simulink model "MdSWReqChk"  (R2024b)
settings: Solver=FixedStepDiscrete  StartTime=0.0  StopTime=10.0  FixedStep=0.01  RelTol=1e-3
undefined symbols (not defined in the file or in its folder): ChkBsyBitArray4s, ChkBsyBitArray6s7s, KeSMSAutoEZEFwdBkwdPosEna_Val, KeSMSuButtonLongPressedThrshldTm_Val, KeSMSuMdNum4s_Val, KeSMSuMdNum6s7s_Val, SetBsyBitArray4s, SetEnBitArray4s
libraries: simulink x16, RspLib x14
(part 1 of 3)
settings Model: Creator=sn2xws  LastModifiedBy=sn55gm
settings Model: ModifiedHistory=|
  | 2023.8.1 CR401790  增加模式21-26的请求
  | V2.1.0
  | 2023.9.18 bug 542961符号方向反了，<= 改为>=
  | V2.3.0
  | 2023.12.28  迎宾向后，条件改为或
  | 2024.7.11 V3.0.0 557模式流程V1.9
  | 2024.8.15 V3.0.1 打断逻辑更新
  | 2024.8.19 V3.0.2 Md30 Md31临时关闭
  | 2024.9.2 V3.0.3 v3.0.1需求共存逻辑更新
  | 2024.9.26 V3.0.4 bsybitall 不使用的模式去除Md8
  | 2024.10.15 V3.0.5 增加Md57 Md58
  | 2024.11.5 V3.0.6 对req做跳变1判断
  | 2024.12.5 V3.0.7 Md8与Md30，md31应可以共存
  | 2024.12.19 V3.0.8 BUG 963441 Md9 与Md11不共存问题
  | 2024.12.19 V3.0.9 BUG 963459 Md53 与Md31不共存问题（NotUsedMode值错误，bsyall不看notusedmode）
  | 2024.12.24 V3.1.0 BUG 964134 VIPALL LUGALL VIPEXITALL模式可以单侧打断，只看剩余运行模式与其他模式共存的逻辑
  | 2024.12.25 V3.1.1 VIPRbsy应增加7sLUGR
  | 25.6.28 V3.13.0 新增大记忆模式MD61 MD62
  | 25.7.11 V3.13.1 md61 md62请求连反
settings SolverCC: AlgebraicLoopSolver=TrustRegion
settings DataIOCC: SaveFormat=StructureWithTime  ReturnWorkspaceOutputs=off
settings OptimizationCC: DefaultParameterBehavior=Inlined  EnhancedBackFolding=on  PassReuseOutputArgsAs=Individual arguments  ZeroExternalMemoryAtStartup=off  ZeroInternalMemoryAtStartup=off  OptimizeBlockOrder=speed  DifferentSizesBufferReuse=on  OptimizationCustomize=off  EfficientTunableParamExpr=on
settings DebuggingCC: ParameterTunabilityLossMsg=error  UnconnectedInputMsg=warning  UnconnectedOutputMsg=warning  UnconnectedLineMsg=warning  ArithmeticOperatorsInVariantConditions=warning
settings ModelReferenceCC: EnableRefExpFcnMdlSchedulingChecks=on  ModelReferenceNumInstancesAllowed=Single
settings SFSimCC: MATLABDynamicMemAlloc=off  CustomCodeUndefinedFunction=UseInterfaceOnly
settings RTWCC: Description=AUTOSAR  SystemTargetFile=autosar.tlc  GenCodeOnly=on  TemplateMakefile=ert_default_tmf  GenerateReport=on  IncludeHyperlinkInReport=on  LaunchReport=on  DataTypeReplacement=CDataTypesFixedWidth  GenerateTraceInfo=on  GenerateTraceReport=on  GenerateTraceReportSl=on  GenerateTraceReportSf=on  GenerateTraceReportEml=on  GenerateCodeMetricsReport=on  GPUComputeCapability=3.5
settings CodeAppCC: ForceParamTrailComments=on  IgnoreCustomStorageClasses=off  OperatorAnnotations=on  SimulinkDataObjDesc=on  SFDataObjDesc=on  InsertBlockDesc=on
settings STFCustomTargetCC: TargetLangStandard=C99 (ISO)  MultiwordLength=256  ParMdlRefBuildCompliant=on  CompOptLevelCompliant=on  IncludeMdlTerminateFcn=off  CombineOutputUpdateFcns=on  SuppressErrorStatus=on  ERTCustomFileBanners=on  SupportNonFinite=off  SupportComplex=off  SupportContinuousTime=off  SupportNonInlinedSFcns=off  RemoveResetFunc=on  MATLABClassNameForMDSCustomization=Simulink.SoftwareTarget.ERTCustomization  AutosarCompliant=on  UseToolchainInfoCompliant=on  LookupTableObjectStructAxisOrder=2,1,3,4,...  LUTObjectStructOrderEvenSpacing=Size,Table,Breakpoints  SystemTargetFile=autosar.tlc
settings ERTTargetCC: TargetLangStandard=C99 (ISO)  ConcurrentExecutionCompliant=off  IncludeMdlTerminateFcn=off  SuppressErrorStatus=on  SupportNonFinite=off  SupportComplex=off  ModelStepFunctionPrototypeControlCompliant=off  CPPClassGenCompliant=off  AutosarCompliant=on  LookupTableObjectStructAxisOrder=2,1,3,4,...  LUTObjectStructOrderEvenSpacing=Size,Table,Breakpoints  ERTCustomFileTemplate=example_file_process.tlc  ERTFilePackagingFormat=Compact  BooleanTrueId=TRUE  BooleanFalseId=FALSE  DynamicArrayContainerType=coder::array

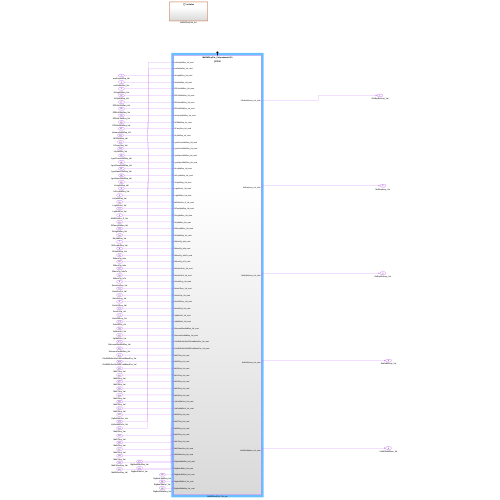
[thumbnail: Simulink's stored preview of the top-level diagram]
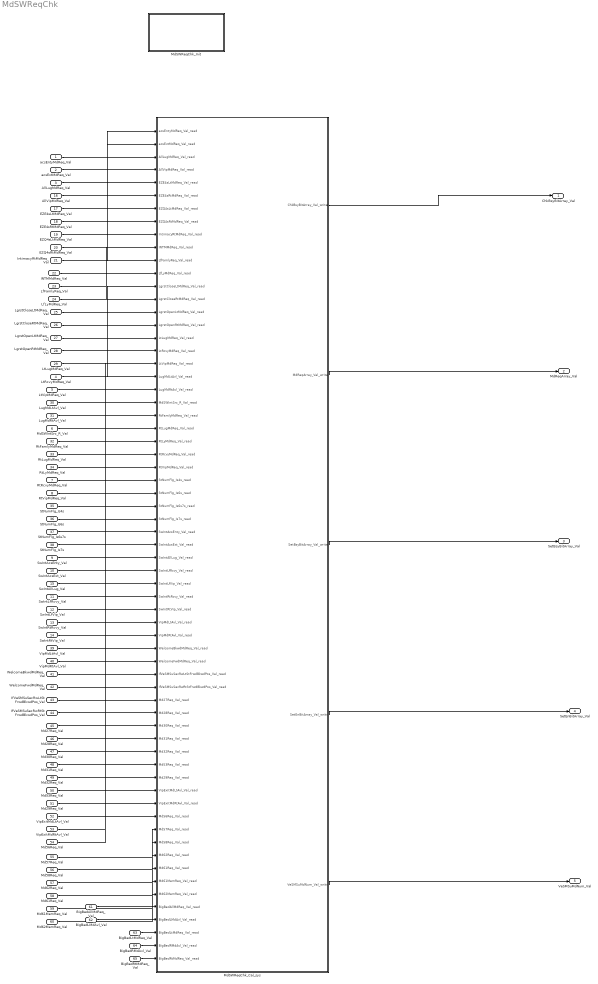
== system MdSWReqChk ==
  acsEntyMdReq_Val : Inport  OutDataTypeStr=boolean  PortDimensions=1
  acsExtMdReq_Val : Inport  Port=2  OutDataTypeStr=boolean  PortDimensions=1
  AllLugMdReq_Val : Inport  Port=3  OutDataTypeStr=boolean  PortDimensions=1
  LtRcvyMdReq_Val : Inport  Port=4  OutDataTypeStr=boolean  PortDimensions=1
  LtVipMdReq_Val : Inport  Port=5  OutDataTypeStr=boolean  PortDimensions=1
  MdSWIntSrc_R_Val : Inport  Port=6  OutDataTypeStr=uint16  PortDimensions=1
  RtRcvyMdReq_Val : Inport  Port=7  OutDataTypeStr=boolean  PortDimensions=1
  RtVipMdReq_Val : Inport  Port=8  OutDataTypeStr=boolean  PortDimensions=1
  SwIntAcsEnty_Val : Inport  Port=9  OutDataTypeStr=IntEnable  PortDimensions=1
  SwIntAcsExt_Val : Inport  Port=10  OutDataTypeStr=IntEnable  PortDimensions=1
  SwIntLfRcvy_Val : Inport  Port=11  OutDataTypeStr=IntEnable  PortDimensions=1
  SwIntLfVip_Val : Inport  Port=12  OutDataTypeStr=IntEnable  PortDimensions=1
  SwIntRtRcvy_Val : Inport  Port=13  OutDataTypeStr=IntEnable  PortDimensions=1
  SwIntRtVip_Val : Inport  Port=14  OutDataTypeStr=IntEnable  PortDimensions=1
  SwIntAllLug_Val : Inport  Port=15  OutDataTypeStr=IntEnable  PortDimensions=1
  AllVipMdReq_Val : Inport  Port=16  OutDataTypeStr=boolean  PortDimensions=1
  EZE4sLtMdReq_Val : Inport  Port=17  OutDataTypeStr=boolean  PortDimensions=1
  EZE4sRtMdReq_Val : Inport  Port=18  OutDataTypeStr=boolean  PortDimensions=1
  EZQ4sLtMdReq_Val : Inport  Port=19  OutDataTypeStr=boolean  PortDimensions=1
  EZQ4sRtMdReq_Val : Inport  Port=20  OutDataTypeStr=boolean  PortDimensions=1
  IntimacyRtMdReq_Val : Inport  Port=21  OutDataTypeStr=boolean  PortDimensions=1
  INTMMdReq_Val : Inport  Port=22  OutDataTypeStr=boolean  PortDimensions=1
  LfFamlyReq_Val : Inport  Port=23  OutDataTypeStr=boolean  PortDimensions=1
  LfLyMdReq_Val : Inport  Port=24  OutDataTypeStr=boolean  PortDimensions=1
  LgrstCloseLtMdReq_Val : Inport  Port=25  OutDataTypeStr=boolean  PortDimensions=1
  LgrstCloseRtMdReq_Val : Inport  Port=26  OutDataTypeStr=boolean  PortDimensions=1
  LgrstOpenLtMdReq_Val : Inport  Port=27  OutDataTypeStr=boolean  PortDimensions=1
  LgrstOpenRtMdReq_Val : Inport  Port=28  OutDataTypeStr=boolean  PortDimensions=1
  LtLugMdReq_Val : Inport  Port=29  OutDataTypeStr=boolean  PortDimensions=1
  LugMdLtAvl_Val : Inport  Port=30  OutDataTypeStr=boolean  PortDimensions=1
  LugMdRtAvl_Val : Inport  Port=31  OutDataTypeStr=boolean  PortDimensions=1
  RtFamlyMdReq_Val : Inport  Port=32  OutDataTypeStr=boolean  PortDimensions=1
  RtLugMdReq_Val : Inport  Port=33  OutDataTypeStr=boolean  PortDimensions=1
  RtLyMdReq_Val : Inport  Port=34  OutDataTypeStr=boolean  PortDimensions=1
  StNumFlg_Is4s : Inport  Port=35  OutDataTypeStr=boolean  PortDimensions=1
  StNumFlg_Is6s : Inport  Port=36  OutDataTypeStr=boolean  PortDimensions=1
  StNumFlg_Is6s7s : Inport  Port=37  OutDataTypeStr=boolean  PortDimensions=1
  StNumFlg_Is7s : Inport  Port=38  OutDataTypeStr=boolean  PortDimensions=1
  VipMdLtAvl_Val : Inport  Port=39  OutDataTypeStr=boolean  PortDimensions=1
  VipMdRtAvl_Val : Inport  Port=40  OutDataTypeStr=boolean  PortDimensions=1
  WelcomeBkwdMdReq_Val : Inport  Port=41  OutDataTypeStr=boolean  PortDimensions=1
  WelcomeFwdMdReq_Val : Inport  Port=42  OutDataTypeStr=boolean  PortDimensions=1
  IfVeSMSuSecRwLtStFrwdBkwdPos_Val : Inport  Port=43  OutDataTypeStr=uint16  PortDimensions=1
  IfVeSMSuSecRwRtStFrwdBkwdPos_Val : Inport  Port=44  OutDataTypeStr=uint16  PortDimensions=1
  Md27Req_Val : Inport  Port=45  OutDataTypeStr=boolean  PortDimensions=1
  Md28Req_Val : Inport  Port=46  OutDataTypeStr=boolean  PortDimensions=1
  Md30Req_Val : Inport  Port=47  OutDataTypeStr=boolean  PortDimensions=1
  Md31Req_Val : Inport  Port=48  OutDataTypeStr=boolean  PortDimensions=1
  Md32Req_Val : Inport  Port=49  OutDataTypeStr=boolean  PortDimensions=1
  Md53Req_Val : Inport  Port=50  OutDataTypeStr=boolean  PortDimensions=1
  Md29Req_Val : Inport  Port=51  OutDataTypeStr=boolean  PortDimensions=1
  VipExitMdLtAvl_Val : Inport  Port=52  OutDataTypeStr=boolean  PortDimensions=1
  VipExitMdRtAvl_Val : Inport  Port=53  OutDataTypeStr=boolean  PortDimensions=1
  Md56Req_Val : Inport  Port=54  OutDataTypeStr=boolean  PortDimensions=1
  Md57Req_Val : Inport  Port=55  OutDataTypeStr=boolean  PortDimensions=1
  Md58Req_Val : Inport  Port=56  OutDataTypeStr=boolean  PortDimensions=1
  Md62Req_Val : Inport  Port=57  OutDataTypeStr=boolean  PortDimensions=1
  Md61Req_Val : Inport  Port=58  OutDataTypeStr=boolean  PortDimensions=1
  Md61MemReq_Val : Inport  Port=59  OutDataTypeStr=boolean  PortDimensions=1
  Md62MemReq_Val : Inport  Port=60  OutDataTypeStr=boolean  PortDimensions=1
  BigBedAllMdReq_Val : Inport  Port=61  OutDataTypeStr=boolean  PortDimensions=1
  BigBedLMdAvl_Val : Inport  Port=62  OutDataTypeStr=boolean  PortDimensions=1
  BigBedLtMdReq_Val : Inport  Port=63  OutDataTypeStr=boolean  PortDimensions=1
  BigBedRMdAvl_Val : Inport  Port=64  OutDataTypeStr=boolean  PortDimensions=1
  BigBedRtMdReq_Val : Inport  Port=65  OutDataTypeStr=boolean  PortDimensions=1
  MdSWReqChk_Cal_sys : Subsystem
  MdSWReqChk_Init : Subsystem
  ChkBsyBitArray_Val : Outport  OutDataTypeStr=uint32  PortDimensions=32  VectorParamsAs1DForOutWhenUnconnected=off
  MdReqArray_Val : Outport  Port=2  OutDataTypeStr=boolean  PortDimensions=32  VectorParamsAs1DForOutWhenUnconnected=off
  SetBsyBitArray_Val : Outport  Port=3  OutDataTypeStr=uint32  PortDimensions=32  VectorParamsAs1DForOutWhenUnconnected=off
  SetEnBitArray_Val : Outport  Port=4  OutDataTypeStr=uint32  PortDimensions=32  VectorParamsAs1DForOutWhenUnconnected=off
  VeSMSuMdNum_Val : Outport  Port=5  OutDataTypeStr=uint8  PortDimensions=1  VectorParamsAs1DForOutWhenUnconnected=off
  wires:
  acsEntyMdReq_Val/1 -> MdSWReqChk_Cal_sys/1(acsEntyMdReq_Val_read)
  acsExtMdReq_Val/1 -> MdSWReqChk_Cal_sys/2(acsExtMdReq_Val_read)
  AllLugMdReq_Val/1 -> MdSWReqChk_Cal_sys/3(AllLugMdReq_Val_read)
  LtRcvyMdReq_Val/1 -> MdSWReqChk_Cal_sys/18(LtRcvyMdReq_Val_read)
  LtVipMdReq_Val/1 -> MdSWReqChk_Cal_sys/19(LtVipMdReq_Val_read)
  MdSWIntSrc_R_Val/1 -> MdSWReqChk_Cal_sys/22(MdSWIntSrc_R_Val_read)
  RtRcvyMdReq_Val/1 -> MdSWReqChk_Cal_sys/26(RtRcvyMdReq_Val_read)
  RtVipMdReq_Val/1 -> MdSWReqChk_Cal_sys/27(RtVipMdReq_Val_read)
  SwIntAcsEnty_Val/1 -> MdSWReqChk_Cal_sys/32(SwIntAcsEnty_Val_read)
  SwIntAcsExt_Val/1 -> MdSWReqChk_Cal_sys/33(SwIntAcsExt_Val_read)
  SwIntLfRcvy_Val/1 -> MdSWReqChk_Cal_sys/35(SwIntLfRcvy_Val_read)
  SwIntLfVip_Val/1 -> MdSWReqChk_Cal_sys/36(SwIntLfVip_Val_read)
  SwIntRtRcvy_Val/1 -> MdSWReqChk_Cal_sys/37(SwIntRtRcvy_Val_read)
  SwIntRtVip_Val/1 -> MdSWReqChk_Cal_sys/38(SwIntRtVip_Val_read)
  SwIntAllLug_Val/1 -> MdSWReqChk_Cal_sys/34(SwIntAllLug_Val_read)
  AllVipMdReq_Val/1 -> MdSWReqChk_Cal_sys/4(AllVipMdReq_Val_read)
  EZE4sLtMdReq_Val/1 -> MdSWReqChk_Cal_sys/5(EZE4sLtMdReq_Val_read)
  EZE4sRtMdReq_Val/1 -> MdSWReqChk_Cal_sys/6(EZE4sRtMdReq_Val_read)
  EZQ4sLtMdReq_Val/1 -> MdSWReqChk_Cal_sys/7(EZQ4sLtMdReq_Val_read)
  EZQ4sRtMdReq_Val/1 -> MdSWReqChk_Cal_sys/8(EZQ4sRtMdReq_Val_read)
  IntimacyRtMdReq_Val/1 -> MdSWReqChk_Cal_sys/9(IntimacyRtMdReq_Val_read)
  INTMMdReq_Val/1 -> MdSWReqChk_Cal_sys/10(INTMMdReq_Val_read)
  LfFamlyReq_Val/1 -> MdSWReqChk_Cal_sys/11(LfFamlyReq_Val_read)
  LfLyMdReq_Val/1 -> MdSWReqChk_Cal_sys/12(LfLyMdReq_Val_read)
  LgrstCloseLtMdReq_Val/1 -> MdSWReqChk_Cal_sys/13(LgrstCloseLtMdReq_Val_read)
  LgrstCloseRtMdReq_Val/1 -> MdSWReqChk_Cal_sys/14(LgrstCloseRtMdReq_Val_read)
  LgrstOpenLtMdReq_Val/1 -> MdSWReqChk_Cal_sys/15(LgrstOpenLtMdReq_Val_read)
  LgrstOpenRtMdReq_Val/1 -> MdSWReqChk_Cal_sys/16(LgrstOpenRtMdReq_Val_read)
  LtLugMdReq_Val/1 -> MdSWReqChk_Cal_sys/17(LtLugMdReq_Val_read)
  LugMdLtAvl_Val/1 -> MdSWReqChk_Cal_sys/20(LugMdLtAvl_Val_read)
  LugMdRtAvl_Val/1 -> MdSWReqChk_Cal_sys/21(LugMdRtAvl_Val_read)
  RtFamlyMdReq_Val/1 -> MdSWReqChk_Cal_sys/23(RtFamlyMdReq_Val_read)
  RtLugMdReq_Val/1 -> MdSWReqChk_Cal_sys/24(RtLugMdReq_Val_read)
  RtLyMdReq_Val/1 -> MdSWReqChk_Cal_sys/25(RtLyMdReq_Val_read)
  StNumFlg_Is4s/1 -> MdSWReqChk_Cal_sys/28(StNumFlg_Is4s_read)
  StNumFlg_Is6s/1 -> MdSWReqChk_Cal_sys/29(StNumFlg_Is6s_read)
  StNumFlg_Is6s7s/1 -> MdSWReqChk_Cal_sys/30(StNumFlg_Is6s7s_read)
  StNumFlg_Is7s/1 -> MdSWReqChk_Cal_sys/31(StNumFlg_Is7s_read)
  VipMdLtAvl_Val/1 -> MdSWReqChk_Cal_sys/39(VipMdLtAvl_Val_read)
  VipMdRtAvl_Val/1 -> MdSWReqChk_Cal_sys/40(VipMdRtAvl_Val_read)
  WelcomeBkwdMdReq_Val/1 -> MdSWReqChk_Cal_sys/41(WelcomeBkwdMdReq_Val_read)
  WelcomeFwdMdReq_Val/1 -> MdSWReqChk_Cal_sys/42(WelcomeFwdMdReq_Val_read)
  MdSWReqChk_Cal_sys/1(ChkBsyBitArray_Val_write) -> ChkBsyBitArray_Val/1
  MdSWReqChk_Cal_sys/2(MdReqArray_Val_write) -> MdReqArray_Val/1
  MdSWReqChk_Cal_sys/3(SetBsyBitArray_Val_write) -> SetBsyBitArray_Val/1
  MdSWReqChk_Cal_sys/4(SetEnBitArray_Val_write) -> SetEnBitArray_Val/1
  MdSWReqChk_Cal_sys/5(VeSMSuMdNum_Val_write) -> VeSMSuMdNum_Val/1
  IfVeSMSuSecRwLtStFrwdBkwdPos_Val/1 -> MdSWReqChk_Cal_sys/43(IfVeSMSuSecRwLtStFrwdBkwdPos_Val_read)
  IfVeSMSuSecRwRtStFrwdBkwdPos_Val/1 -> MdSWReqChk_Cal_sys/44(IfVeSMSuSecRwRtStFrwdBkwdPos_Val_read)
  Md27Req_Val/1 -> MdSWReqChk_Cal_sys/45(Md27Req_Val_read)
  Md28Req_Val/1 -> MdSWReqChk_Cal_sys/46(Md28Req_Val_read)
  Md30Req_Val/1 -> MdSWReqChk_Cal_sys/47(Md30Req_Val_read)
  Md31Req_Val/1 -> MdSWReqChk_Cal_sys/48(Md31Req_Val_read)
  Md32Req_Val/1 -> MdSWReqChk_Cal_sys/49(Md32Req_Val_read)
  Md53Req_Val/1 -> MdSWReqChk_Cal_sys/50(Md53Req_Val_read)
  Md29Req_Val/1 -> MdSWReqChk_Cal_sys/51(Md29Req_Val_read)
  VipExitMdLtAvl_Val/1 -> MdSWReqChk_Cal_sys/52(VipExitMdLtAvl_Val_read)
  VipExitMdRtAvl_Val/1 -> MdSWReqChk_Cal_sys/53(VipExitMdRtAvl_Val_read)
  Md56Req_Val/1 -> MdSWReqChk_Cal_sys/54(Md56Req_Val_read)
  Md57Req_Val/1 -> MdSWReqChk_Cal_sys/55(Md57Req_Val_read)
  Md58Req_Val/1 -> MdSWReqChk_Cal_sys/56(Md58Req_Val_read)
  Md62Req_Val/1 -> MdSWReqChk_Cal_sys/57(Md62Req_Val_read)
  Md61Req_Val/1 -> MdSWReqChk_Cal_sys/58(Md61Req_Val_read)
  Md61MemReq_Val/1 -> MdSWReqChk_Cal_sys/59(Md61MemReq_Val_read)
  Md62MemReq_Val/1 -> MdSWReqChk_Cal_sys/60(Md62MemReq_Val_read)
  BigBedAllMdReq_Val/1 -> MdSWReqChk_Cal_sys/61(BigBedAllMdReq_Val_read)
  BigBedLMdAvl_Val/1 -> MdSWReqChk_Cal_sys/62(BigBedLMdAvl_Val_read)
  BigBedLtMdReq_Val/1 -> MdSWReqChk_Cal_sys/63(BigBedLtMdReq_Val_read)
  BigBedRMdAvl_Val/1 -> MdSWReqChk_Cal_sys/64(BigBedRMdAvl_Val_read)
  BigBedRtMdReq_Val/1 -> MdSWReqChk_Cal_sys/65(BigBedRtMdReq_Val_read)

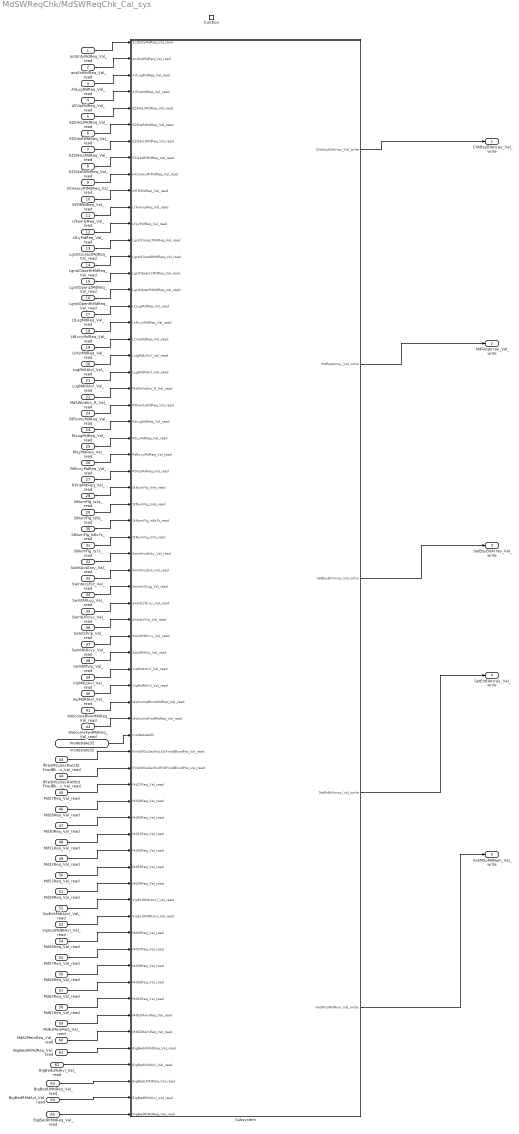
== system MdSWReqChk/MdSWReqChk_Cal_sys ==
  acsEntyMdReq_Val_read : Inport
  acsExtMdReq_Val_read : Inport  Port=2
  AllLugMdReq_Val_read : Inport  Port=3
  AllVipMdReq_Val_read : Inport  Port=4
  EZE4sLtMdReq_Val_read : Inport  Port=5
  EZE4sRtMdReq_Val_read : Inport  Port=6
  EZQ4sLtMdReq_Val_read : Inport  Port=7
  EZQ4sRtMdReq_Val_read : Inport  Port=8
  IntimacyRtMdReq_Val_read : Inport  Port=9
  INTMMdReq_Val_read : Inport  Port=10
  LfFamlyReq_Val_read : Inport  Port=11
  LfLyMdReq_Val_read : Inport  Port=12
  LgrstCloseLtMdReq_Val_read : Inport  Port=13
  LgrstCloseRtMdReq_Val_read : Inport  Port=14
  LgrstOpenLtMdReq_Val_read : Inport  Port=15
  LgrstOpenRtMdReq_Val_read : Inport  Port=16
  LtLugMdReq_Val_read : Inport  Port=17
  LtRcvyMdReq_Val_read : Inport  Port=18
  LtVipMdReq_Val_read : Inport  Port=19
  LugMdLtAvl_Val_read : Inport  Port=20
  LugMdRtAvl_Val_read : Inport  Port=21
  MdSWIntSrc_R_Val_read : Inport  Port=22
  RtFamlyMdReq_Val_read : Inport  Port=23
  RtLugMdReq_Val_read : Inport  Port=24
  RtLyMdReq_Val_read : Inport  Port=25
  RtRcvyMdReq_Val_read : Inport  Port=26
  RtVipMdReq_Val_read : Inport  Port=27
  StNumFlg_Is4s_read : Inport  Port=28
  StNumFlg_Is6s_read : Inport  Port=29
  StNumFlg_Is6s7s_read : Inport  Port=30
  StNumFlg_Is7s_read : Inport  Port=31
  SwIntAcsEnty_Val_read : Inport  Port=32
  SwIntAcsExt_Val_read : Inport  Port=33
  SwIntAllLug_Val_read : Inport  Port=34
  SwIntLfRcvy_Val_read : Inport  Port=35
  SwIntLfVip_Val_read : Inport  Port=36
  SwIntRtRcvy_Val_read : Inport  Port=37
  SwIntRtVip_Val_read : Inport  Port=38
  VipMdLtAvl_Val_read : Inport  Port=39
  VipMdRtAvl_Val_read : Inport  Port=40
  WelcomeBkwdMdReq_Val_read : Inport  Port=41
  WelcomeFwdMdReq_Val_read : Inport  Port=42
  IfVeSMSuSecRwLtStFrwdBkwdPos_Val_read : Inport  Port=43
  IfVeSMSuSecRwRtStFrwdBkwdPos_Val_read : Inport  Port=44
  Md27Req_Val_read : Inport  Port=45
  Md28Req_Val_read : Inport  Port=46
  Md30Req_Val_read : Inport  Port=47
  Md31Req_Val_read : Inport  Port=48
  Md32Req_Val_read : Inport  Port=49
  Md53Req_Val_read : Inport  Port=50
  Md29Req_Val_read : Inport  Port=51
  VipExitMdLtAvl_Val_read : Inport  Port=52
  VipExitMdRtAvl_Val_read : Inport  Port=53
  Md56Req_Val_read : Inport  Port=54
  Md57Req_Val_read : Inport  Port=55
  Md58Req_Val_read : Inport  Port=56
  Md62Req_Val_read : Inport  Port=57
  Md61Req_Val_read : Inport  Port=58
  Md61MemReq_Val_read : Inport  Port=59
  Md62MemReq_Val_read : Inport  Port=60
  BigBedAllMdReq_Val_read : Inport  Port=61
  BigBedLMdAvl_Val_read : Inport  Port=62
  BigBedLtMdReq_Val_read : Inport  Port=63
  BigBedRMdAvl_Val_read : Inport  Port=64
  BigBedRtMdReq_Val_read : Inport  Port=65
  function : TriggerPort  TriggerType=function-call  IsSimulinkFunction=on  FunctionName=MdSWReqChk_Cal  VariantControl=(inherit)
  Subsystem : Subsystem
  modestate32 : ArgIn  OutDataTypeStr=uint32  ArgumentName=modestate32
  ChkBsyBitArray_Val_write : Outport  VectorParamsAs1DForOutWhenUnconnected=off
      settings: EnsureOutportIsVirtual=on
  MdReqArray_Val_write : Outport  Port=2  VectorParamsAs1DForOutWhenUnconnected=off
      settings: EnsureOutportIsVirtual=on
  SetBsyBitArray_Val_write : Outport  Port=3  VectorParamsAs1DForOutWhenUnconnected=off
      settings: EnsureOutportIsVirtual=on
  SetEnBitArray_Val_write : Outport  Port=4  VectorParamsAs1DForOutWhenUnconnected=off
      settings: EnsureOutportIsVirtual=on
  VeSMSuMdNum_Val_write : Outport  Port=5  VectorParamsAs1DForOutWhenUnconnected=off
      settings: EnsureOutportIsVirtual=on
  wires:
  acsEntyMdReq_Val_read/1 -> Subsystem/1(acsEntyMdReq_Val_read)
  acsExtMdReq_Val_read/1 -> Subsystem/2(acsExtMdReq_Val_read)
  AllLugMdReq_Val_read/1 -> Subsystem/3(AllLugMdReq_Val_read)
  AllVipMdReq_Val_read/1 -> Subsystem/4(AllVipMdReq_Val_read)
  EZE4sLtMdReq_Val_read/1 -> Subsystem/5(EZE4sLtMdReq_Val_read)
  EZE4sRtMdReq_Val_read/1 -> Subsystem/6(EZE4sRtMdReq_Val_read)
  EZQ4sLtMdReq_Val_read/1 -> Subsystem/7(EZQ4sLtMdReq_Val_read)
  EZQ4sRtMdReq_Val_read/1 -> Subsystem/8(EZQ4sRtMdReq_Val_read)
  IntimacyRtMdReq_Val_read/1 -> Subsystem/9(IntimacyRtMdReq_Val_read)
  INTMMdReq_Val_read/1 -> Subsystem/10(INTMMdReq_Val_read)
  LfFamlyReq_Val_read/1 -> Subsystem/11(LfFamlyReq_Val_read)
  LfLyMdReq_Val_read/1 -> Subsystem/12(LfLyMdReq_Val_read)
  LgrstCloseLtMdReq_Val_read/1 -> Subsystem/13(LgrstCloseLtMdReq_Val_read)
  LgrstCloseRtMdReq_Val_read/1 -> Subsystem/14(LgrstCloseRtMdReq_Val_read)
  LgrstOpenLtMdReq_Val_read/1 -> Subsystem/15(LgrstOpenLtMdReq_Val_read)
  LgrstOpenRtMdReq_Val_read/1 -> Subsystem/16(LgrstOpenRtMdReq_Val_read)
  LtLugMdReq_Val_read/1 -> Subsystem/17(LtLugMdReq_Val_read)
  LtRcvyMdReq_Val_read/1 -> Subsystem/18(LtRcvyMdReq_Val_read)
  LtVipMdReq_Val_read/1 -> Subsystem/19(LtVipMdReq_Val_read)
  LugMdLtAvl_Val_read/1 -> Subsystem/20(LugMdLtAvl_Val_read)
  LugMdRtAvl_Val_read/1 -> Subsystem/21(LugMdRtAvl_Val_read)
  MdSWIntSrc_R_Val_read/1 -> Subsystem/22(MdSWIntSrc_R_Val_read)
  RtFamlyMdReq_Val_read/1 -> Subsystem/23(RtFamlyMdReq_Val_read)
  RtLugMdReq_Val_read/1 -> Subsystem/24(RtLugMdReq_Val_read)
  RtLyMdReq_Val_read/1 -> Subsystem/25(RtLyMdReq_Val_read)
  RtRcvyMdReq_Val_read/1 -> Subsystem/26(RtRcvyMdReq_Val_read)
  RtVipMdReq_Val_read/1 -> Subsystem/27(RtVipMdReq_Val_read)
  StNumFlg_Is4s_read/1 -> Subsystem/28(StNumFlg_Is4s_read)
  StNumFlg_Is6s_read/1 -> Subsystem/29(StNumFlg_Is6s_read)
  StNumFlg_Is6s7s_read/1 -> Subsystem/30(StNumFlg_Is6s7s_read)
  StNumFlg_Is7s_read/1 -> Subsystem/31(StNumFlg_Is7s_read)
  SwIntAcsEnty_Val_read/1 -> Subsystem/32(SwIntAcsEnty_Val_read)
  SwIntAcsExt_Val_read/1 -> Subsystem/33(SwIntAcsExt_Val_read)
  SwIntAllLug_Val_read/1 -> Subsystem/34(SwIntAllLug_Val_read)
  SwIntLfRcvy_Val_read/1 -> Subsystem/35(SwIntLfRcvy_Val_read)
  SwIntLfVip_Val_read/1 -> Subsystem/36(SwIntLfVip_Val_read)
  SwIntRtRcvy_Val_read/1 -> Subsystem/37(SwIntRtRcvy_Val_read)
  SwIntRtVip_Val_read/1 -> Subsystem/38(SwIntRtVip_Val_read)
  VipMdLtAvl_Val_read/1 -> Subsystem/39(VipMdLtAvl_Val_read)
  VipMdRtAvl_Val_read/1 -> Subsystem/40(VipMdRtAvl_Val_read)
  WelcomeBkwdMdReq_Val_read/1 -> Subsystem/41(WelcomeBkwdMdReq_Val_read)
  WelcomeFwdMdReq_Val_read/1 -> Subsystem/42(WelcomeFwdMdReq_Val_read)
  Subsystem/1(ChkBsyBitArray_Val_write) -> ChkBsyBitArray_Val_write/1
  Subsystem/2(MdReqArray_Val_write) -> MdReqArray_Val_write/1
  Subsystem/3(SetBsyBitArray_Val_write) -> SetBsyBitArray_Val_write/1
  Subsystem/4(SetEnBitArray_Val_write) -> SetEnBitArray_Val_write/1
  modestate32/1 -> Subsystem/43(modestate32)
  Subsystem/5(VeSMSuMdNum_Val_write) -> VeSMSuMdNum_Val_write/1
  IfVeSMSuSecRwLtStFrwdBkwdPos_Val_read/1 -> Subsystem/44(IfVeSMSuSecRwLtStFrwdBkwdPos_Val_read)
  IfVeSMSuSecRwRtStFrwdBkwdPos_Val_read/1 -> Subsystem/45(IfVeSMSuSecRwRtStFrwdBkwdPos_Val_read)
  Md27Req_Val_read/1 -> Subsystem/46(Md27Req_Val_read)
  Md28Req_Val_read/1 -> Subsystem/47(Md28Req_Val_read)
  Md30Req_Val_read/1 -> Subsystem/48(Md30Req_Val_read)
  Md31Req_Val_read/1 -> Subsystem/49(Md31Req_Val_read)
  Md32Req_Val_read/1 -> Subsystem/50(Md32Req_Val_read)
  Md53Req_Val_read/1 -> Subsystem/51(Md53Req_Val_read)
  Md29Req_Val_read/1 -> Subsystem/52(Md29Req_Val_read)
  VipExitMdLtAvl_Val_read/1 -> Subsystem/53(VipExitMdLtAvl_Val_read)
  VipExitMdRtAvl_Val_read/1 -> Subsystem/54(VipExitMdRtAvl_Val_read)
  Md56Req_Val_read/1 -> Subsystem/55(Md56Req_Val_read)
  Md57Req_Val_read/1 -> Subsystem/56(Md57Req_Val_read)
  Md58Req_Val_read/1 -> Subsystem/57(Md58Req_Val_read)
  Md62Req_Val_read/1 -> Subsystem/58(Md62Req_Val_read)
  Md61Req_Val_read/1 -> Subsystem/59(Md61Req_Val_read)
  Md61MemReq_Val_read/1 -> Subsystem/60(Md61MemReq_Val_read)
  Md62MemReq_Val_read/1 -> Subsystem/61(Md62MemReq_Val_read)
  BigBedAllMdReq_Val_read/1 -> Subsystem/62(BigBedAllMdReq_Val_read)
  BigBedLMdAvl_Val_read/1 -> Subsystem/63(BigBedLMdAvl_Val_read)
  BigBedLtMdReq_Val_read/1 -> Subsystem/64(BigBedLtMdReq_Val_read)
  BigBedRMdAvl_Val_read/1 -> Subsystem/65(BigBedRMdAvl_Val_read)
  BigBedRtMdReq_Val_read/1 -> Subsystem/66(BigBedRtMdReq_Val_read)

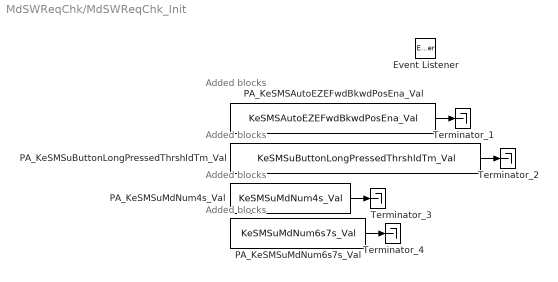
== system MdSWReqChk/MdSWReqChk_Init ==
  note: Added blocks
  note: Added blocks
  note: Added blocks
  note: Added blocks
  Event Listener : EventListener  EventName=reset
  PA_KeSMSAutoEZEFwdBkwdPosEna_Val : Constant  Value=KeSMSAutoEZEFwdBkwdPosEna_Val
  PA_KeSMSuButtonLongPressedThrshldTm_Val : Constant  Value=KeSMSuButtonLongPressedThrshldTm_Val
  PA_KeSMSuMdNum4s_Val : Constant  Value=KeSMSuMdNum4s_Val
  PA_KeSMSuMdNum6s7s_Val : Constant  Value=KeSMSuMdNum6s7s_Val
  Terminator_{1..4} (4 alike) : Terminator
  wires:
  PA_KeSMSAutoEZEFwdBkwdPosEna_Val/1 -> Terminator_1/1
  PA_KeSMSuButtonLongPressedThrshldTm_Val/1 -> Terminator_2/1
  PA_KeSMSuMdNum4s_Val/1 -> Terminator_3/1
  PA_KeSMSuMdNum6s7s_Val/1 -> Terminator_4/1
